simulink model "2_ESM_NonLinear"  (R2016a)
settings: Solver=ode1  StartTime=0.0  StopTime=150  FixedStep=0.001  RelTol=1e-3
values from neighbouring files (symbols this model uses):
  C = 1.3    [2_ESM_Parameters.m]    (also in 3_ZSM_Parameters.m)
  c_h = c_h * 180 / pi    (= 143239.448783)    [2_ESM_Parameters.m]    (also in 3_ZSM_Parameters.m)
  c_v = c_v * 180 / pi    (= 78109.773598)    [2_ESM_Parameters.m]    (also in 3_ZSM_Parameters.m)
  E = 0.85    [2_ESM_Parameters.m]    (also in 3_ZSM_Parameters.m)
  F_x_max = m_v * 9.81 * mu    (= 6619.9842)    [3_ZSM_Parameters.m]
  F_x_min = - F_x_max    (= -6619.9842)    [3_ZSM_Parameters.m]
  m_h = 750.0    (= 750)    [2_ESM_Parameters.m]    (also in 3_ZSM_Parameters.m)
  m_v = 749.8    [2_ESM_Parameters.m]    (also in 3_ZSM_Parameters.m)
  Mode_Tire = setting(i,6)    [2_ESM_Parameters.m]    (also in 3_ZSM_Parameters.m = 2-i)
  mu = 0.9    [2_ESM_Parameters.m]    (also in 3_ZSM_Parameters.m)
  psi_p_init = 0    [2_ESM_Parameters.m]    (also in 3_ZSM_Parameters.m = 0.0416666666667)
  T_R = Test(:,3)    [3_ZSM_Parameters.m]
  T_t = Test(:,1)    [3_ZSM_Parameters.m]
  T_v = Test(:,2)    [3_ZSM_Parameters.m]
undefined symbols (not defined in the file): l_h, l_v, Lenkwinkel, m, Radlenkwinkel, T_z
libraries: simulink x2
settings Model: Creator=KFZ00  LastModifiedBy=Mario
settings DataIOCC: SaveFormat=Array  SaveOutput=off  TimeSaveName=t_out
settings DebuggingCC: AllowSymbolicDim=off
settings ModelReferenceCC: PropagateSignalLabelsOutOfModel=off
settings GRTTargetCC: GeneratePreprocessorConditionals=Use local settings

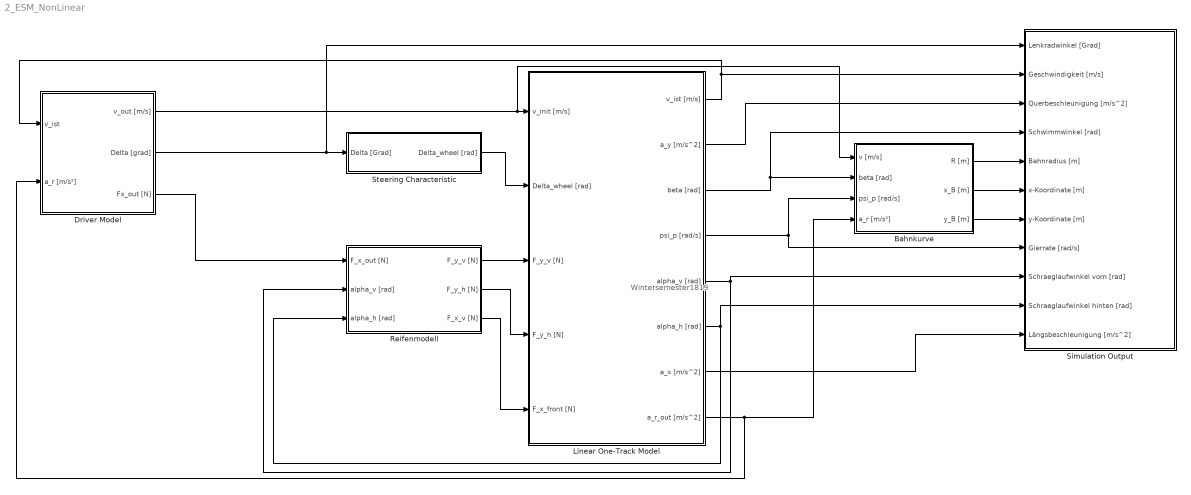
== system 2_ESM_NonLinear ==
  note: Wintersemester1819
  Bahnkurve : Subsystem
  Driver Model : Subsystem
  Linear One-Track Model : Subsystem  mask(Vehicle Model){m_body=m, l_front=l_v, l_rear=l_h, I_zz_body=T_z}
      mask prompts: m_body "Vehicle Body Mass [kg]"; l_front "Distance COG Front Axle [m]"; l_rear "Distance COG Rear Axle [m]"; I_zz_body "Vehicle Body Intertia zz [kgm^2]"
      mask help:
      | One-track model.
      |
      | Source for equations:
      | Von Vietinghoff, A.: Nichtlineare Regelung von Kraftfahrzeugen in
      | querdynamisch kritischen Fahrsituationen. Dissertation, Universität
      | Karlsruhe, S. 10 - 33, 2008.
  Reifenmodell : Subsystem
  Simulation Output : Subsystem
  Steering Characteristic : Subsystem  mask(Steering Model){Input_values=Lenkwinkel, Steering_angles=Radlenkwinkel}
      mask prompts: Input_values "Steering Input Values [°]"; Steering_angles "Wheel Steer Angles [°]"
      mask help:
      | Steering model uses a look-up table to determine the current wheel
      | steer angle.
      | The steering angle of the rear wheel is set to zero!
      |
      | In order to configure the look-up table define the input values (steering
      | wheel angle in °) and the corresponding wheel steer angles (in °).
  wires:
  Linear One-Track Model/6(alpha_h [rad]) -> Simulation Output/10(Schraeglaufwinkel hinten [rad]), Reifenmodell/3(alpha_h [rad])
  Linear One-Track Model/5(alpha_v [rad]) -> Simulation Output/9(Schraeglaufwinkel vorn [rad]), Reifenmodell/2(alpha_v [rad])
  Steering Characteristic/1(Delta_wheel [rad]) -> Linear One-Track Model/2(Delta_wheel [rad])
  Linear One-Track Model/3(beta [rad]) -> Simulation Output/4(Schwimmwinkel [rad]), Bahnkurve/2(beta [rad])
  Linear One-Track Model/2(a_y [m/s^2]) -> Simulation Output/3(Querbeschleunigung [m/s^2])
  Bahnkurve/2(x_B [m]) -> Simulation Output/6(x-Koordinate [m])
  Bahnkurve/1(R [m]) -> Simulation Output/5(Bahnradius [m])
  Bahnkurve/3(y_B [m]) -> Simulation Output/7(y-Koordinate [m])
  Linear One-Track Model/4(psi_p [rad/s]) -> Simulation Output/8(Gierrate [rad/s]), Bahnkurve/3(psi_p [rad/s])
  Linear One-Track Model/7(a_x [m/s^2]) -> Simulation Output/11(Längsbeschleunigung [m/s^2])
  Driver Model/2(Delta [grad]) -> Simulation Output/1(Lenkradwinkel [Grad]), Steering Characteristic/1(Delta [Grad])
  Driver Model/1(v_out [m/s]) -> Bahnkurve/1(v [m/s]), Linear One-Track Model/1(v_init [m/s])
  Driver Model/3(Fx_out [N]) -> Reifenmodell/1(F_x_out [N])
  Reifenmodell/1(F_y_v [N]) -> Linear One-Track Model/3(F_y_v [N])
  Reifenmodell/2(F_y_h [N]) -> Linear One-Track Model/4(F_y_h [N])
  Reifenmodell/3(F_x_v [N]) -> Linear One-Track Model/5(F_x_front [N])
  Linear One-Track Model/1(v_ist [m/s]) -> Driver Model/1(v_ist), Simulation Output/2(Geschwindigkeit [m/s])
  Linear One-Track Model/8(a_r_out [m/s^2]) -> Driver Model/2(a_r [m/s²]), Bahnkurve/4(a_r [m/s²])

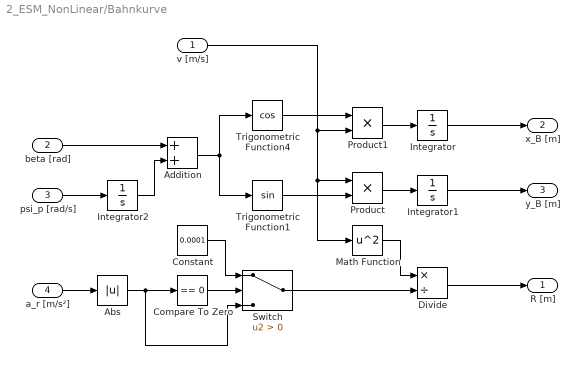
== system 2_ESM_NonLinear/Bahnkurve ==
  v [m/s] : Inport
  beta [rad] : Inport  Port=2
  psi_p [rad/s] : Inport  Port=3
  a_r [m/s²] : Inport  Port=4
  Abs : Abs
  Addition : Sum
  Compare To Zero : simulink/Logic and Bit Operations/Compare To Zero  relop===  OutDataTypeStr=boolean
  Constant : Constant  Value=0.0001
  Divide : Product  Inputs=*/
  Integrator : Integrator
  Integrator1 : Integrator
  Integrator2 : Integrator
  Math Function : Math  Operator=square  SaturateOnIntegerOverflow=on
  Product : Product
  Product1 : Product
  Switch : Switch  Criteria=u2 > Threshold
  Trigonometric Function1 : Trigonometry
  Trigonometric Function4 : Trigonometry  Operator=cos
  R [m] : Outport
  x_B [m] : Outport  Port=2
  y_B [m] : Outport  Port=3
  wires:
  Trigonometric Function4/1 -> Product1/1
  Trigonometric Function1/1 -> Product/2
  Product/1 -> Integrator1/1
  Addition/1 -> Trigonometric Function1/1, Trigonometric Function4/1
  psi_p [rad/s]/1 -> Integrator2/1
  Integrator2/1 -> Addition/2
  Product1/1 -> Integrator/1
  Integrator/1 -> x_B [m]/1
  Integrator1/1 -> y_B [m]/1
  beta [rad]/1 -> Addition/1
  Switch/1 -> Divide/2
  Compare To Zero/1 -> Switch/2
  Divide/1 -> R [m]/1
  Constant/1 -> Switch/1
  Abs/1 -> Switch/3, Compare To Zero/1
  v [m/s]/1 -> Math Function/1, Product/1, Product1/2
  Math Function/1 -> Divide/1
  a_r [m/s²]/1 -> Abs/1

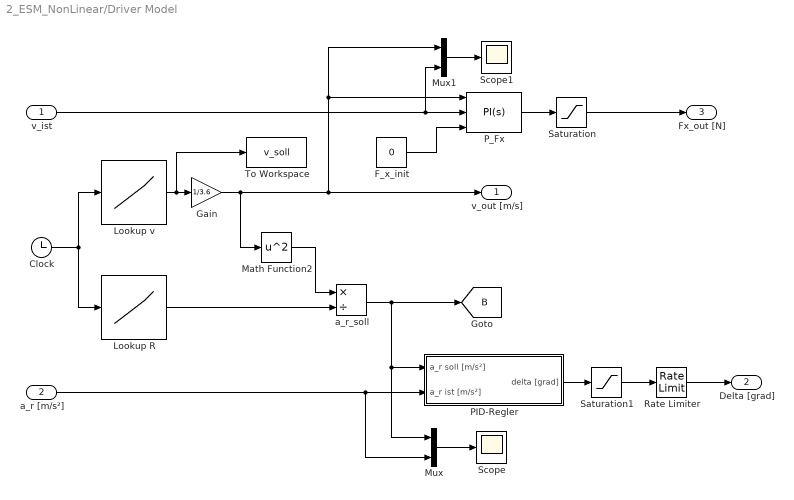
== system 2_ESM_NonLinear/Driver Model ==
  v_ist : Inport
  a_r [m/s²] : Inport  Port=2
  Clock : Clock
  F_x_init : Constant  Value=0
  Gain : Gain  Gain=1/3.6
  Lookup R : Lookup_n-D  NumberOfTableDimensions=1  BreakpointsForDimension1=T_t  Table=T_R  InternalRulePriority=Speed  RndMeth=Simplest  InputSameDT=on
  Lookup v : Lookup_n-D  NumberOfTableDimensions=1  BreakpointsForDimension1=T_t  Table=T_v  InternalRulePriority=Speed  RndMeth=Simplest  InputSameDT=on
  Math Function2 : Math  Operator=square  SaturateOnIntegerOverflow=on
  Mux : Mux  Inputs=2
  Mux1 : Mux  Inputs=2
  PID-Regler : Subsystem
  P_Fx : simulink/Continuous/PID Controller (2DOF)  Controller=PI  TimeDomain=Continuous-time  SampleTime=-1  IntegratorMethod=Forward Euler  FilterMethod=Forward Euler  Form=Parallel  UseFilter=on  ControllerParametersSource=internal  P=10000  I=0  D=0  N=100  b=1  c=1  InitialConditionSource=external  InitialConditionForIntegrator=0  InitialConditionForFilter=0  ExternalReset=none  LimitOutput=off  UpperSaturationLimit=9000  LowerSaturationLimit=0  LinearizeAsGain=on  AntiWindupMode=none  Kb=1  TrackingMode=off  Kt=1  PParamMin=[]  PParamMax=[]  IParamMin=[]  IParamMax=[]  DParamMin=[]  DParamMax=[]  NParamMin=[]  NParamMax=[]  bParamMin=[]  bParamMax=[]  cParamMin=[]  cParamMax=[]  KbParamMin=[]  KbParamMax=[]  KtParamMin=[]  KtParamMax=[]  POutMin=[]  POutMax=[]  IOutMin=[]  IOutMax=[]  DOutMin=[]  DOutMax=[]  NOutMin=[]  NOutMax=[]  bOutMin=[]  bOutMax=[]  cOutMin=[]  cOutMax=[]  KbOutMin=[]  KbOutMax=[]  KtOutMin=[]  KtOutMax=[]  IntegratorOutMin=[]  IntegratorOutMax=[]  FilterOutMin=[]  FilterOutMax=[]  SumOutMin=[]  SumOutMax=[]  Sum1OutMin=[]  Sum1OutMax=[]  Sum2OutMin=[]  Sum2OutMax=[]  Sum3OutMin=[]  Sum3OutMax=[]  SumI1OutMin=[]  SumI1OutMax=[]  SumI2OutMin=[]  SumI2OutMax=[]  SumI3OutMin=[]  SumI3OutMax=[]  SumDOutMin=[]  SumDOutMax=[]  SaturationOutMin=[]  SaturationOutMax=[]  IntegratorContinuousStateAttributes=''  IntegratorStateMustResolveToSignalObject=off  IntegratorRTWStateStorageClass=Auto  FilterContinuousStateAttributes=''  FilterStateMustResolveToSignalObject=off  FilterRTWStateStorageClass=Auto  DifferentiatorICPrevScaledInput=0  DifferentiatorOutMin=[]  DifferentiatorOutMax=[]
  Rate Limiter : RateLimiter  RisingSlewLimit=600  FallingSlewLimit=-600  SampleTimeMode=inherited
  Saturation : Saturate  UpperLimit=F_x_max  LowerLimit=F_x_min
  Saturation1 : Saturate  UpperLimit=410  LowerLimit=-405
  Scope : Scope
  Scope1 : Scope
  To Workspace : ToWorkspace  VariableName=v_soll  SampleTime=-1
      settings: Save2DSignal=2-D array (concatenate along first dimension)
  a_r_soll : Product  Inputs=*/
  v_out [m/s] : Outport
  Delta [grad] : Outport  Port=2
  Fx_out [N] : Outport  Port=3
  tag scope: B=global
  wires:
  Lookup v/1 -> To Workspace/1, Gain/1
  Clock/1 -> Lookup v/1, Lookup R/1
  Mux/1 -> Scope/1
  Mux1/1 -> Scope1/1
  Gain/1 -> P_Fx/1, Mux1/1, v_out [m/s]/1, Math Function2/1
  v_ist/1 -> Mux1/2, P_Fx/2
  Saturation/1 -> Fx_out [N]/1
  F_x_init/1 -> P_Fx/3
  Math Function2/1 -> a_r_soll/1
  P_Fx/1 -> Saturation/1
  a_r_soll/1 -> Mux/1, PID-Regler/1(a_r soll [m/s²]), [B]
  Lookup R/1 -> a_r_soll/2
  PID-Regler/1(delta [grad]) -> Saturation1/1
  Saturation1/1 -> Rate Limiter/1
  Rate Limiter/1 -> Delta [grad]/1
  a_r [m/s²]/1 -> PID-Regler/2(a_r ist [m/s²]), Mux/2

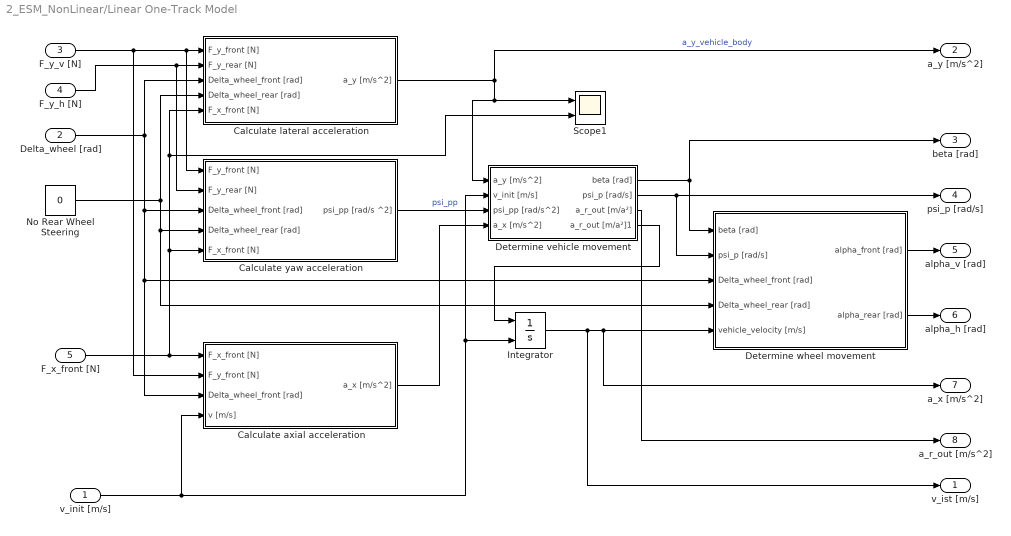
== system 2_ESM_NonLinear/Linear One-Track Model ==
  v_init [m/s] : Inport  OutDataTypeStr=double
  Delta_wheel [rad] : Inport  Port=2  OutDataTypeStr=double
  F_y_v [N] : Inport  Port=3  OutDataTypeStr=double
  F_y_h [N] : Inport  Port=4  OutDataTypeStr=double
  F_x_front [N] : Inport  Port=5  OutDataTypeStr=double
  Calculate axial acceleration : Subsystem
  Calculate lateral acceleration : Subsystem
  Calculate yaw acceleration : Subsystem
  Determine vehicle movement : Subsystem
  Determine wheel movement : Subsystem
  Integrator : Integrator  InitialConditionSource=external
  No Rear Wheel Steering : Constant  Value=0
  Scope1 : Scope  NumInputPorts=2
  v_ist [m/s] : Outport  OutDataTypeStr=double
  a_y [m/s^2] : Outport  Port=2  OutDataTypeStr=double
  beta [rad] : Outport  Port=3  OutDataTypeStr=double
  psi_p [rad/s] : Outport  Port=4  OutDataTypeStr=double
  alpha_v [rad] : Outport  Port=5  OutDataTypeStr=double
  alpha_h [rad] : Outport  Port=6  OutDataTypeStr=double
  a_x [m/s^2] : Outport  Port=7  OutDataTypeStr=double
  a_r_out [m/s^2] : Outport  Port=8  OutDataTypeStr=double
  wires:
  Determine wheel movement/2(alpha_rear [rad]) -> alpha_h [rad]/1
  Determine wheel movement/1(alpha_front [rad]) -> alpha_v [rad]/1
  Determine vehicle movement/1(beta [rad]) -> beta [rad]/1, Determine wheel movement/1(beta [rad])
  Calculate yaw acceleration/1(psi_pp [rad/s ^2]) -> Determine vehicle movement/3(psi_pp [rad/s^2])  "psi_pp"
  Calculate lateral acceleration/1(a_y [m/s^2]) -> Scope1/1, Determine vehicle movement/1(a_y [m/s^2]), a_y [m/s^2]/1  "a_y_vehicle_body"
  F_y_v [N]/1 -> Calculate axial acceleration/2(F_y_front [N]), Calculate yaw acceleration/1(F_y_front [N]), Calculate lateral acceleration/1(F_y_front [N])
  F_y_h [N]/1 -> Calculate yaw acceleration/2(F_y_rear [N]), Calculate lateral acceleration/2(F_y_rear [N])
  No Rear Wheel Steering/1 -> Determine wheel movement/4(Delta_wheel_rear [rad]), Calculate yaw acceleration/4(Delta_wheel_rear [rad]), Calculate lateral acceleration/4(Delta_wheel_rear [rad])
  Delta_wheel [rad]/1 -> Calculate axial acceleration/3(Delta_wheel_front [rad]), Determine wheel movement/3(Delta_wheel_front [rad]), Calculate yaw acceleration/3(Delta_wheel_front [rad]), Calculate lateral acceleration/3(Delta_wheel_front [rad])
  F_x_front [N]/1 -> Calculate axial acceleration/1(F_x_front [N]), Scope1/2, Calculate lateral acceleration/5(F_x_front [N]), Calculate yaw acceleration/5(F_x_front [N])
  Determine vehicle movement/3(a_r_out [m/a²]) -> a_r_out [m/s^2]/1
  Determine vehicle movement/2(psi_p [rad/s]) -> Determine wheel movement/2(psi_p [rad/s]), psi_p [rad/s]/1
  v_init [m/s]/1 -> Calculate axial acceleration/4(v [m/s]), Integrator/2, Determine vehicle movement/2(v_init [m/s])
  Calculate axial acceleration/1(a_x [m/s^2]) -> Determine vehicle movement/4(a_x [m/s^2])
  Integrator/1 -> v_ist [m/s]/1, a_x [m/s^2]/1, Determine wheel movement/5(vehicle_velocity [m/s])
  Determine vehicle movement/4(a_r_out [m/a²]1) -> Integrator/1

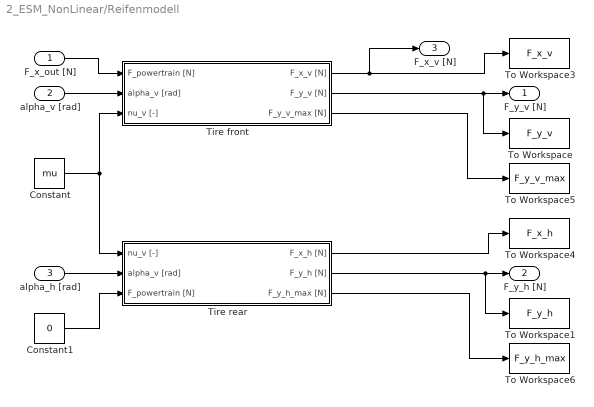
== system 2_ESM_NonLinear/Reifenmodell ==
  F_x_out [N] : Inport
  alpha_v [rad] : Inport  Port=2
  alpha_h [rad] : Inport  Port=3
  Constant : Constant  Value=mu
  Constant1 : Constant  Value=0
  Tire front : Subsystem
  Tire rear : Subsystem
  To Workspace : ToWorkspace  VariableName=F_y_v  SampleTime=-1
      settings: Save2DSignal=2-D array (concatenate along first dimension)
  To Workspace1 : ToWorkspace  VariableName=F_y_h  SampleTime=-1
      settings: Save2DSignal=2-D array (concatenate along first dimension)
  To Workspace3 : ToWorkspace  VariableName=F_x_v  SampleTime=-1
      settings: Save2DSignal=2-D array (concatenate along first dimension)
  To Workspace4 : ToWorkspace  VariableName=F_x_h  SampleTime=-1
      settings: Save2DSignal=2-D array (concatenate along first dimension)
  To Workspace5 : ToWorkspace  VariableName=F_y_v_max  SampleTime=-1
      settings: Save2DSignal=2-D array (concatenate along first dimension)
  To Workspace6 : ToWorkspace  VariableName=F_y_h_max  SampleTime=-1
      settings: Save2DSignal=2-D array (concatenate along first dimension)
  F_y_v [N] : Outport
  F_y_h [N] : Outport  Port=2
  F_x_v [N] : Outport  Port=3
  wires:
  F_x_out [N]/1 -> Tire front/1(F_powertrain [N])
  alpha_v [rad]/1 -> Tire front/2(alpha_v [rad])
  Constant/1 -> Tire front/3(nu_v [-]), Tire rear/1(nu_v [-])
  alpha_h [rad]/1 -> Tire rear/2(alpha_v [rad])
  Tire front/2(F_y_v [N]) -> To Workspace/1, F_y_v [N]/1
  Tire rear/2(F_y_h [N]) -> To Workspace1/1, F_y_h [N]/1
  Tire front/1(F_x_v [N]) -> F_x_v [N]/1, To Workspace3/1
  Tire rear/1(F_x_h [N]) -> To Workspace4/1
  Tire front/3(F_y_v_max [N]) -> To Workspace5/1
  Tire rear/3(F_y_h_max [N]) -> To Workspace6/1
  Constant1/1 -> Tire rear/3(F_powertrain [N])

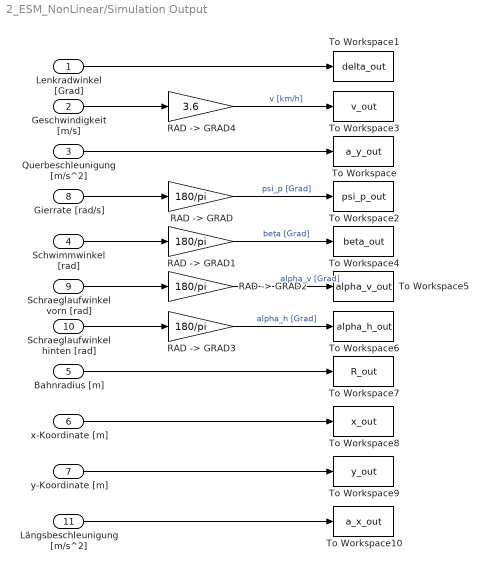
== system 2_ESM_NonLinear/Simulation Output ==
  Lenkradwinkel [Grad] : Inport
  Geschwindigkeit [m/s] : Inport  Port=2
  Querbeschleunigung [m/s^2] : Inport  Port=3
  Schwimmwinkel [rad] : Inport  Port=4
  Bahnradius [m] : Inport  Port=5
  x-Koordinate [m] : Inport  Port=6
  y-Koordinate [m] : Inport  Port=7
  Gierrate [rad/s] : Inport  Port=8
  Schraeglaufwinkel vorn [rad] : Inport  Port=9
  Schraeglaufwinkel hinten [rad] : Inport  Port=10
  Längsbeschleunigung [m/s^2] : Inport  Port=11
  RAD -> GRAD{,1..3} (4 alike) : Gain  Gain=180/pi
  "RAD -> GRAD4" : Gain  Gain=3.6
  To Workspace : ToWorkspace  VariableName=a_y_out  SampleTime=-1
      settings: Save2DSignal=2-D array (concatenate along first dimension)
  To Workspace1 : ToWorkspace  VariableName=delta_out  SampleTime=-1
      settings: Save2DSignal=2-D array (concatenate along first dimension)
  To Workspace10 : ToWorkspace  VariableName=a_x_out  SampleTime=-1
      settings: Save2DSignal=2-D array (concatenate along first dimension)
  To Workspace2 : ToWorkspace  VariableName=psi_p_out  SampleTime=-1
      settings: Save2DSignal=2-D array (concatenate along first dimension)
  To Workspace3 : ToWorkspace  VariableName=v_out  SampleTime=-1
      settings: Save2DSignal=2-D array (concatenate along first dimension)
  To Workspace4 : ToWorkspace  VariableName=beta_out  SampleTime=-1
      settings: Save2DSignal=2-D array (concatenate along first dimension)
  To Workspace5 : ToWorkspace  VariableName=alpha_v_out  SampleTime=-1
      settings: Save2DSignal=2-D array (concatenate along first dimension)
  To Workspace6 : ToWorkspace  VariableName=alpha_h_out  SampleTime=-1
      settings: Save2DSignal=2-D array (concatenate along first dimension)
  To Workspace7 : ToWorkspace  VariableName=R_out  SampleTime=-1
      settings: Save2DSignal=2-D array (concatenate along first dimension)
  To Workspace8 : ToWorkspace  VariableName=x_out  SampleTime=-1
      settings: Save2DSignal=2-D array (concatenate along first dimension)
  To Workspace9 : ToWorkspace  VariableName=y_out  SampleTime=-1
      settings: Save2DSignal=2-D array (concatenate along first dimension)
  wires:
  Gierrate [rad/s]/1 -> "RAD -> GRAD"/1
  "RAD -> GRAD"/1 -> To Workspace2/1  "psi_p [Grad]"
  Lenkradwinkel [Grad]/1 -> To Workspace1/1
  Querbeschleunigung [m/s^2]/1 -> To Workspace/1
  Geschwindigkeit [m/s]/1 -> "RAD -> GRAD4"/1
  Schwimmwinkel [rad]/1 -> "RAD -> GRAD1"/1
  "RAD -> GRAD1"/1 -> To Workspace4/1  "beta [Grad]"
  Schraeglaufwinkel vorn [rad]/1 -> "RAD -> GRAD2"/1
  "RAD -> GRAD2"/1 -> To Workspace5/1  "alpha_v [Grad]"
  Schraeglaufwinkel hinten [rad]/1 -> "RAD -> GRAD3"/1
  "RAD -> GRAD3"/1 -> To Workspace6/1  "alpha_h [Grad]"
  Bahnradius [m]/1 -> To Workspace7/1
  x-Koordinate [m]/1 -> To Workspace8/1
  y-Koordinate [m]/1 -> To Workspace9/1
  "RAD -> GRAD4"/1 -> To Workspace3/1  "v [km/h]"
  Längsbeschleunigung [m/s^2]/1 -> To Workspace10/1

== system 2_ESM_NonLinear/Steering Characteristic ==
  Delta [Grad] : Inport  OutDataTypeStr=double
  1-D Lookup Table : Lookup_n-D  NumberOfTableDimensions=1  BreakpointsForDimension1=Input_values  Table=Steering_angles  InternalRulePriority=Speed  RndMeth=Simplest  InputSameDT=on
  "Grad -> RAD1" : Gain  Gain=pi/180
  Delta_wheel [rad] : Outport  OutDataTypeStr=double
  wires:
  Delta [Grad]/1 -> 1-D Lookup Table/1
  1-D Lookup Table/1 -> "Grad -> RAD1"/1
  "Grad -> RAD1"/1 -> Delta_wheel [rad]/1

== system 2_ESM_NonLinear/Driver Model/PID-Regler ==
  note: Regelabweichung
  a_r soll [m/s²] : Inport
  a_r ist [m/s²] : Inport  Port=2
  Add : Sum  Inputs=+++
  Derivative : Derivative
  Integrator : Integrator
  Kd : Gain  Gain=0.002376
  Ki : Gain  Gain=9900
  Kp : Gain  Gain=9.9
  Sum1 : Sum  Inputs=|+-
  To Workspace : ToWorkspace  VariableName=a_r_soll  SampleTime=-1
      settings: Save2DSignal=2-D array (concatenate along first dimension)
  To Workspace1 : ToWorkspace  VariableName=a_r_ist  SampleTime=-1
      settings: Save2DSignal=2-D array (concatenate along first dimension)
  delta [grad] : Outport
  wires:
  a_r ist [m/s²]/1 -> To Workspace1/1, Sum1/2
  Integrator/1 -> Add/2
  a_r soll [m/s²]/1 -> To Workspace/1, Sum1/1
  Derivative/1 -> Add/3
  Kp/1 -> Add/1
  Ki/1 -> Integrator/1
  Kd/1 -> Derivative/1
  Sum1/1 -> Kd/1, Kp/1, Ki/1  "e"
  Add/1 -> delta [grad]/1

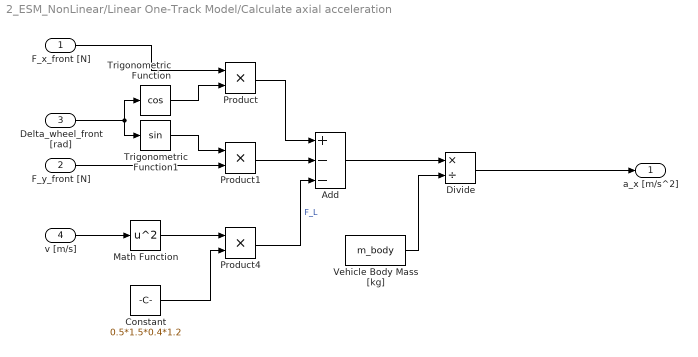
== system 2_ESM_NonLinear/Linear One-Track Model/Calculate axial acceleration ==
  F_x_front [N] : Inport
  F_y_front [N] : Inport  Port=2
  Delta_wheel_front [rad] : Inport  Port=3
  v [m/s] : Inport  Port=4
  Add : Sum  Inputs=+--
  Constant : Constant  Value=0.5*1.5*0.4*1.2
  Divide : Product  Inputs=*/
  Math Function : Math  Operator=square  SaturateOnIntegerOverflow=on
  Product : Product
  Product1 : Product
  Product4 : Product
  Trigonometric Function : Trigonometry  Operator=cos
  Trigonometric Function1 : Trigonometry
  Vehicle Body Mass [kg] : Constant  Value=m_body
  a_x [m/s^2] : Outport
  wires:
  Vehicle Body Mass [kg]/1 -> Divide/2
  Add/1 -> Divide/1
  Product/1 -> Add/1
  Trigonometric Function/1 -> Product/2
  F_x_front [N]/1 -> Product/1
  Delta_wheel_front [rad]/1 -> Trigonometric Function/1, Trigonometric Function1/1
  Product1/1 -> Add/2
  Divide/1 -> a_x [m/s^2]/1
  Product4/1 -> Add/3  "F_L"
  v [m/s]/1 -> Math Function/1
  Constant/1 -> Product4/2
  Math Function/1 -> Product4/1
  Trigonometric Function1/1 -> Product1/1
  F_y_front [N]/1 -> Product1/2

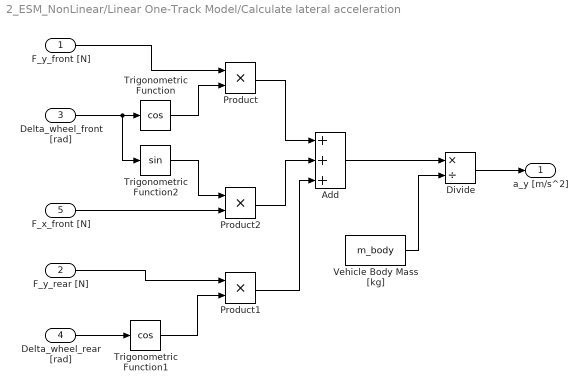
== system 2_ESM_NonLinear/Linear One-Track Model/Calculate lateral acceleration ==
  F_y_front [N] : Inport
  F_y_rear [N] : Inport  Port=2
  Delta_wheel_front [rad] : Inport  Port=3
  Delta_wheel_rear [rad] : Inport  Port=4
  F_x_front [N] : Inport  Port=5
  Add : Sum  Inputs=+++
  Divide : Product  Inputs=*/
  Product : Product
  Product1 : Product
  Product2 : Product
  Trigonometric Function : Trigonometry  Operator=cos
  Trigonometric Function1 : Trigonometry  Operator=cos
  Trigonometric Function2 : Trigonometry
  Vehicle Body Mass [kg] : Constant  Value=m_body
  a_y [m/s^2] : Outport
  wires:
  Divide/1 -> a_y [m/s^2]/1
  Vehicle Body Mass [kg]/1 -> Divide/2
  Add/1 -> Divide/1
  Product/1 -> Add/1
  Trigonometric Function1/1 -> Product1/2
  F_y_rear [N]/1 -> Product1/1
  Trigonometric Function/1 -> Product/2
  F_y_front [N]/1 -> Product/1
  Delta_wheel_rear [rad]/1 -> Trigonometric Function1/1
  Delta_wheel_front [rad]/1 -> Trigonometric Function2/1, Trigonometric Function/1
  Trigonometric Function2/1 -> Product2/1
  F_x_front [N]/1 -> Product2/2
  Product2/1 -> Add/2
  Product1/1 -> Add/3

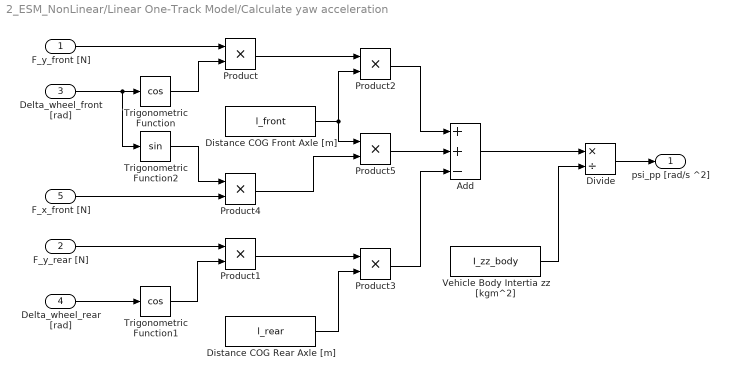
== system 2_ESM_NonLinear/Linear One-Track Model/Calculate yaw acceleration ==
  F_y_front [N] : Inport
  F_y_rear [N] : Inport  Port=2
  Delta_wheel_front [rad] : Inport  Port=3
  Delta_wheel_rear [rad] : Inport  Port=4
  F_x_front [N] : Inport  Port=5
  Add : Sum  Inputs=++-
  Distance COG Front Axle [m] : Constant  Value=l_front
  Distance COG Rear Axle [m] : Constant  Value=l_rear
  Divide : Product  Inputs=*/
  Product{,1..5} (6 alike) : Product
  Trigonometric Function : Trigonometry  Operator=cos
  Trigonometric Function1 : Trigonometry  Operator=cos
  Trigonometric Function2 : Trigonometry
  Vehicle Body Intertia zz [kgm^2] : Constant  Value=I_zz_body
  psi_pp [rad/s ^2] : Outport
  wires:
  Product1/1 -> Product3/1
  Distance COG Rear Axle [m]/1 -> Product3/2
  Product2/1 -> Add/1
  Product/1 -> Product2/1
  Divide/1 -> psi_pp [rad/s ^2]/1
  Vehicle Body Intertia zz [kgm^2]/1 -> Divide/2
  Add/1 -> Divide/1
  Trigonometric Function1/1 -> Product1/2
  F_y_rear [N]/1 -> Product1/1
  Trigonometric Function/1 -> Product/2
  F_y_front [N]/1 -> Product/1
  Delta_wheel_rear [rad]/1 -> Trigonometric Function1/1
  Delta_wheel_front [rad]/1 -> Trigonometric Function2/1, Trigonometric Function/1
  Trigonometric Function2/1 -> Product4/1
  F_x_front [N]/1 -> Product4/2
  Product3/1 -> Add/3
  Distance COG Front Axle [m]/1 -> Product2/2, Product5/1
  Product4/1 -> Product5/2
  Product5/1 -> Add/2

== system 2_ESM_NonLinear/Linear One-Track Model/Determine vehicle movement ==
  a_y [m/s^2] : Inport
  v_init [m/s] : Inport  Port=2
  psi_pp [rad/s^2] : Inport  Port=3
  a_x [m/s^2] : Inport  Port=4
  Calculate radial acceleration : Subsystem
  Constant : Constant  Value=psi_p_init
  Integrator : Integrator  InitialConditionSource=external
  Integrator1 : Integrator  InitialConditionSource=external  InitialCondition=30/3.6
  Integrator3 : Integrator
  Product1 : Product  Inputs=*/  RndMeth=Zero
  Subtract1 : Sum  Inputs=+-
  beta [rad] : Outport
  psi_p [rad/s] : Outport  Port=2
  a_r_out [m/a²] : Outport  Port=3
  a_r_out [m/a²]1 : Outport  Port=4
  wires:
  Product1/1 -> Subtract1/1  "Course angle velocity [rad/s]"
  Integrator3/1 -> Calculate radial acceleration/1(beta [rad]), beta [rad]/1
  Subtract1/1 -> Integrator3/1  "Side slip angle velocity [rad/s]"
  psi_pp [rad/s^2]/1 -> Integrator/1
  Integrator/1 -> Subtract1/2, psi_p [rad/s]/1  "yaw angle velocity [rad/s]"
  Calculate radial acceleration/1(a_r [m/s^2]) -> a_r_out [m/a²]/1, Product1/1
  a_y [m/s^2]/1 -> Calculate radial acceleration/2(a_y [m/s^2])
  a_x [m/s^2]/1 -> Calculate radial acceleration/3(a_x [m/s^2])
  Calculate radial acceleration/2(a_t [m/s^2]) -> a_r_out [m/a²]1/1, Integrator1/1
  Integrator1/1 -> Product1/2
  v_init [m/s]/1 -> Integrator1/2
  Constant/1 -> Integrator/2

== system 2_ESM_NonLinear/Linear One-Track Model/Determine wheel movement ==
  beta [rad] : Inport
  psi_p [rad/s] : Inport  Port=2
  Delta_wheel_front [rad] : Inport  Port=3
  Delta_wheel_rear [rad] : Inport  Port=4
  vehicle_velocity [m/s] : Inport  Port=5
  Distance COG Front Axle [m] : Constant  Value=l_front
  Distance COG Rear Axle [m] : Constant  Value=l_rear
  Math Function : Math  Operator=reciprocal  SaturateOnIntegerOverflow=on
  Product1 : Product  Inputs=3  SaturateOnIntegerOverflow=on  OutDataTypeStr=Inherit: Same as first input
  Product2 : Product  Inputs=3  SaturateOnIntegerOverflow=on  OutDataTypeStr=Inherit: Same as first input
  Sum : Sum  Inputs=+--  SaturateOnIntegerOverflow=on
  Sum1 : Sum  Inputs=+-+  SaturateOnIntegerOverflow=on
  alpha_front [rad] : Outport
  alpha_rear [rad] : Outport  Port=2
  wires:
  Delta_wheel_rear [rad]/1 -> Sum1/3
  Product2/1 -> Sum1/1
  Distance COG Rear Axle [m]/1 -> Product2/3
  Sum1/1 -> alpha_rear [rad]/1
  Sum/1 -> alpha_front [rad]/1
  Product1/1 -> Sum/3
  Math Function/1 -> Product2/1, Product1/3
  vehicle_velocity [m/s]/1 -> Math Function/1
  psi_p [rad/s]/1 -> Product2/2, Product1/2
  Distance COG Front Axle [m]/1 -> Product1/1
  beta [rad]/1 -> Sum1/2, Sum/2
  Delta_wheel_front [rad]/1 -> Sum/1

== system 2_ESM_NonLinear/Reifenmodell/Tire front ==
  F_powertrain [N] : Inport
  alpha_v [rad] : Inport  Port=2
  nu_v [-] : Inport  Port=3
  Constant3 : Constant  Value=m_v*9.81
  Kammscher Kreis : Subsystem
  Pacejka Front Left : Subsystem
  Scope : Scope  NumInputPorts=2
  F_x_v [N] : Outport
  F_y_v [N] : Outport  Port=2
  F_y_v_max [N] : Outport  Port=3
  wires:
  alpha_v [rad]/1 -> Pacejka Front Left/1(alpha_v_in [rad])
  nu_v [-]/1 -> Pacejka Front Left/2(nu_v [-]), Kammscher Kreis/2(nu_v [-])
  Constant3/1 -> Pacejka Front Left/3(F_z_v [N]), Kammscher Kreis/1(F_z_v [N])
  F_powertrain [N]/1 -> Kammscher Kreis/3(F_x_v [N]), F_x_v [N]/1  "F_x_v [N]"
  Pacejka Front Left/1(F_y_v [N]) -> Scope/1, F_y_v [N]/1
  Kammscher Kreis/1(F_y_v_max [N]) -> Pacejka Front Left/4(F_y_v_max [N]), Scope/2, F_y_v_max [N]/1  "F_y_v_max [N]"

== system 2_ESM_NonLinear/Reifenmodell/Tire rear ==
  nu_v [-] : Inport
  alpha_v [rad] : Inport  Port=2
  F_powertrain [N] : Inport  Port=3
  Constant3 : Constant  Value=m_h*9.81
  Kammscher Kreis : Subsystem
  Pacejka Front Left : Subsystem
  Scope : Scope  NumInputPorts=2
  F_x_h [N] : Outport
  F_y_h [N] : Outport  Port=2
  F_y_h_max [N] : Outport  Port=3
  wires:
  alpha_v [rad]/1 -> Pacejka Front Left/1(alpha_h_in [rad])
  nu_v [-]/1 -> Pacejka Front Left/2(nu_h [-]), Kammscher Kreis/2(nu_h [-])
  Constant3/1 -> Pacejka Front Left/3(F_z_h [N]), Kammscher Kreis/1(F_z_h [N])
  F_powertrain [N]/1 -> Kammscher Kreis/3(F_x_h [N]), F_x_h [N]/1  "F_x_h [N]"
  Pacejka Front Left/1(F_y_h [N]) -> Scope/1, F_y_h [N]/1
  Kammscher Kreis/1(F_y_h_max [N]) -> Pacejka Front Left/4(F_y_h_max [N]), Scope/2, F_y_h_max [N]/1  "F_y_v_max [N]"

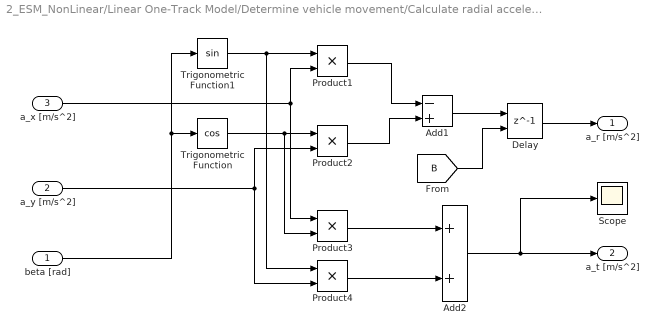
== system 2_ESM_NonLinear/Linear One-Track Model/Determine vehicle movement/Calculate radial acceleration ==
  beta [rad] : Inport
  a_y [m/s^2] : Inport  Port=2
  a_x [m/s^2] : Inport  Port=3
  Add1 : Sum  Inputs=-+
  Add2 : Sum
  Delay : Delay  DelayLength=1  InitialConditionSource=Input port
      settings: InputPortMap=u0,p4
  Product{1..4} (4 alike) : Product
  Scope : Scope
  Trigonometric Function : Trigonometry  Operator=cos
  Trigonometric Function1 : Trigonometry
  a_r [m/s^2] : Outport
  a_t [m/s^2] : Outport  Port=2
  wires:
  Trigonometric Function1/1 -> Product4/1, Product1/1
  Trigonometric Function/1 -> Product3/2, Product2/1
  Product1/1 -> Add1/1
  Product2/1 -> Add1/2
  beta [rad]/1 -> Trigonometric Function/1, Trigonometric Function1/1
  a_x [m/s^2]/1 -> Product3/1, Product1/2
  a_y [m/s^2]/1 -> Product2/2, Product4/2
  Product3/1 -> Add2/1
  Product4/1 -> Add2/2
  Add2/1 -> Scope/1, a_t [m/s^2]/1
  Add1/1 -> Delay/1
  Delay/1 -> a_r [m/s^2]/1
  [B] -> Delay/2

== system 2_ESM_NonLinear/Reifenmodell/Tire front/Kammscher Kreis ==
  F_z_v [N] : Inport
  nu_v [-] : Inport  Port=2
  F_x_v [N] : Inport  Port=3
  Add : Sum  Inputs=+-
  Constant : Constant  Value=Mode_Tire
  Math Function : Math  Operator=square  SaturateOnIntegerOverflow=on
  Math Function1 : Math  Operator=square  SaturateOnIntegerOverflow=on
  Product : Product
  Scope : Scope  NumInputPorts=2
  Sqrt : Sqrt  SaturateOnIntegerOverflow=on
  Switch : Switch  Criteria=u2 > Threshold
  To Workspace3 : ToWorkspace  VariableName=F_v_max  SampleTime=-1
      settings: Save2DSignal=2-D array (concatenate along first dimension)
  F_y_v_max [N] : Outport
  wires:
  Math Function/1 -> Add/2
  Math Function1/1 -> Add/1
  F_z_v [N]/1 -> Product/2  "F_z_v"
  F_x_v [N]/1 -> Math Function/1
  Add/1 -> Sqrt/1  "F_y_max"
  Switch/1 -> F_y_v_max [N]/1
  nu_v [-]/1 -> Product/1
  Sqrt/1 -> Scope/2, Switch/3
  Product/1 -> To Workspace3/1, Scope/1, Switch/1, Math Function1/1
  Constant/1 -> Switch/2

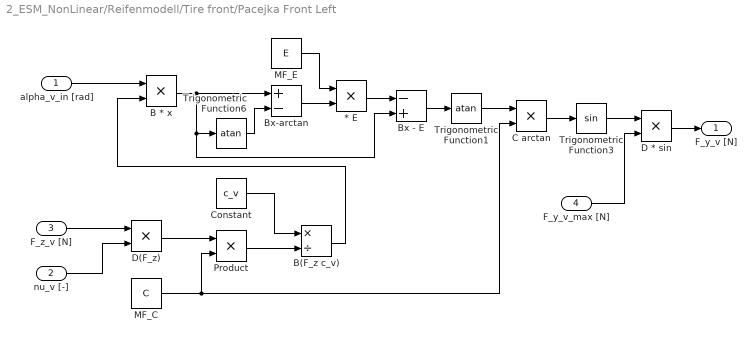
== system 2_ESM_NonLinear/Reifenmodell/Tire front/Pacejka Front Left ==
  alpha_v_in [rad] : Inport
  nu_v [-] : Inport  Port=2
  F_z_v [N] : Inport  Port=3
  F_y_v_max [N] : Inport  Port=4
  * E : Product
  B * x : Product
  B(F_z c_v) : Product  Inputs=*/
  Bx - E : Sum  Inputs=-+
  Bx-arctan : Sum  Inputs=+-
  C arctan : Product
  Constant : Constant  Value=c_v
  D * sin : Product
  D(F_z) : Product
  MF_C : Constant  Value=C
  MF_E : Constant  Value=E
  Product : Product
  Trigonometric Function1 : Trigonometry  Operator=atan
  Trigonometric Function3 : Trigonometry
  Trigonometric Function6 : Trigonometry  Operator=atan
  F_y_v [N] : Outport
  wires:
  D * sin/1 -> F_y_v [N]/1
  Trigonometric Function6/1 -> Bx-arctan/2
  C arctan/1 -> Trigonometric Function3/1
  B * x/1 -> Bx-arctan/1, Bx - E/2, Trigonometric Function6/1
  Bx - E/1 -> Trigonometric Function1/1
  Bx-arctan/1 -> * E/2
  MF_E/1 -> * E/1
  * E/1 -> Bx - E/1
  F_z_v [N]/1 -> D(F_z)/1
  nu_v [-]/1 -> D(F_z)/2
  Product/1 -> B(F_z c_v)/2
  Constant/1 -> B(F_z c_v)/1
  D(F_z)/1 -> Product/1
  MF_C/1 -> C arctan/2, Product/2
  B(F_z c_v)/1 -> B * x/2
  Trigonometric Function1/1 -> C arctan/1
  Trigonometric Function3/1 -> D * sin/1
  alpha_v_in [rad]/1 -> B * x/1
  F_y_v_max [N]/1 -> D * sin/2

== system 2_ESM_NonLinear/Reifenmodell/Tire rear/Kammscher Kreis ==
  F_z_h [N] : Inport
  nu_h [-] : Inport  Port=2
  F_x_h [N] : Inport  Port=3
  Add : Sum  Inputs=+-
  Constant : Constant  Value=Mode_Tire
  Math Function : Math  Operator=square  SaturateOnIntegerOverflow=on
  Math Function1 : Math  Operator=square  SaturateOnIntegerOverflow=on
  Product : Product
  Scope : Scope  NumInputPorts=2
  Sqrt : Sqrt  SaturateOnIntegerOverflow=on
  Switch : Switch  Criteria=u2 > Threshold
  F_y_h_max [N] : Outport
  wires:
  Math Function/1 -> Add/2
  Math Function1/1 -> Add/1
  F_z_h [N]/1 -> Product/2  "F_z_v"
  F_x_h [N]/1 -> Math Function/1
  Add/1 -> Sqrt/1  "F_y_max"
  Switch/1 -> F_y_h_max [N]/1
  nu_h [-]/1 -> Product/1
  Sqrt/1 -> Scope/2, Switch/3
  Product/1 -> Math Function1/1, Scope/1, Switch/1
  Constant/1 -> Switch/2

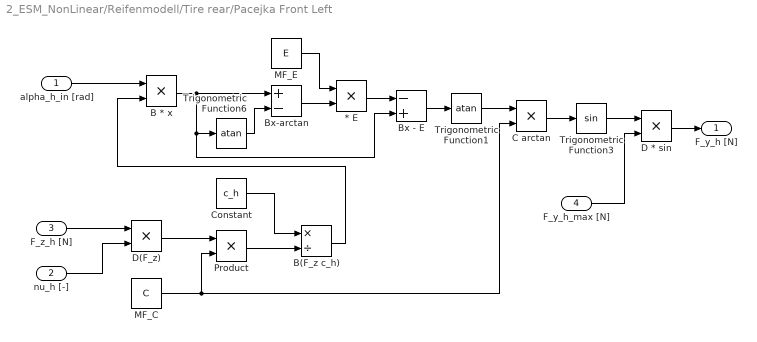
== system 2_ESM_NonLinear/Reifenmodell/Tire rear/Pacejka Front Left ==
  alpha_h_in [rad] : Inport
  nu_h [-] : Inport  Port=2
  F_z_h [N] : Inport  Port=3
  F_y_h_max [N] : Inport  Port=4
  * E : Product
  B * x : Product
  B(F_z c_h) : Product  Inputs=*/
  Bx - E : Sum  Inputs=-+
  Bx-arctan : Sum  Inputs=+-
  C arctan : Product
  Constant : Constant  Value=c_h
  D * sin : Product
  D(F_z) : Product
  MF_C : Constant  Value=C
  MF_E : Constant  Value=E
  Product : Product
  Trigonometric Function1 : Trigonometry  Operator=atan
  Trigonometric Function3 : Trigonometry
  Trigonometric Function6 : Trigonometry  Operator=atan
  F_y_h [N] : Outport
  wires:
  D * sin/1 -> F_y_h [N]/1
  Trigonometric Function6/1 -> Bx-arctan/2
  C arctan/1 -> Trigonometric Function3/1
  B * x/1 -> Bx-arctan/1, Bx - E/2, Trigonometric Function6/1
  Bx - E/1 -> Trigonometric Function1/1
  Bx-arctan/1 -> * E/2
  MF_E/1 -> * E/1
  * E/1 -> Bx - E/1
  F_z_h [N]/1 -> D(F_z)/1
  nu_h [-]/1 -> D(F_z)/2
  Product/1 -> B(F_z c_h)/2
  Constant/1 -> B(F_z c_h)/1
  D(F_z)/1 -> Product/1
  MF_C/1 -> C arctan/2, Product/2
  B(F_z c_h)/1 -> B * x/2
  Trigonometric Function1/1 -> C arctan/1
  Trigonometric Function3/1 -> D * sin/1
  alpha_h_in [rad]/1 -> B * x/1
  F_y_h_max [N]/1 -> D * sin/2
